simulink library "EHP_lib"  (Simulink 7.4)
settings: Solver=FixedStepDiscrete  StartTime=0.0  StopTime=Inf  FixedStep=0.001  RelTol=1e-3
values from neighbouring files (symbols this model uses):
  EHPc_BatIsoTestCmd = mpt.Parameter    [EHP_CAL.m]
  EHPc_r_ClcnRo = mpt.Parameter    [EHP_CAL.m]
  EHPc_r_IsoDiagInitVal = mpt.Parameter    [EHP_CAL.m]
undefined symbols (not defined in the file or in its folder): BCU_Drive_St, BCU_FastCharge_St, BCU_SlowCharge_St
libraries: Defined_Functionality x12, simulink x4
settings Model: Creator=yanlijuan2  LastModifiedBy=sunsijun

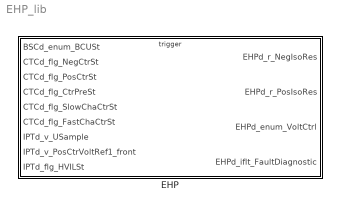
== system EHP_lib ==
  EHP : Subsystem  TreatAsAtomicUnit=on

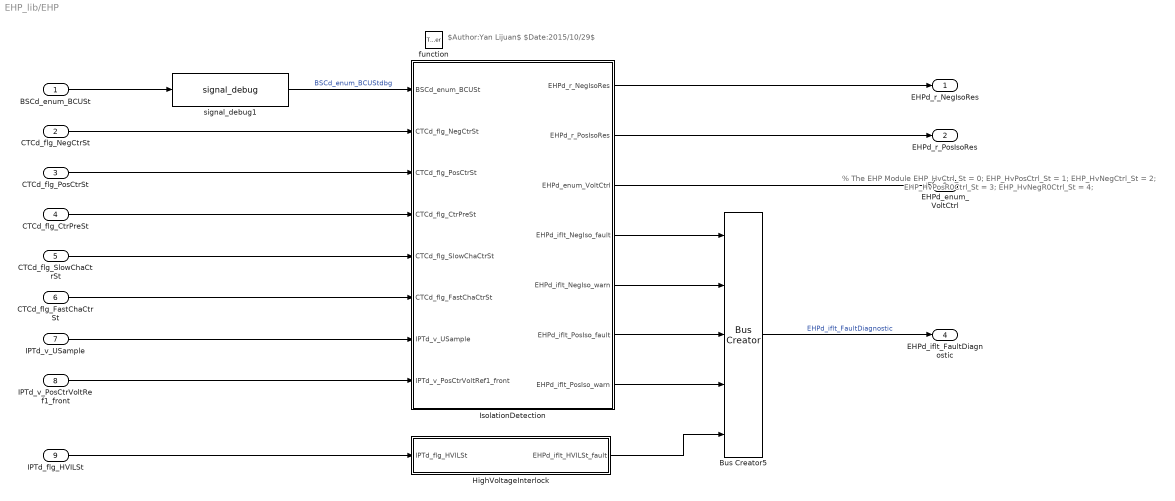
== system EHP_lib/EHP ==
  note: % The EHP Module
      | EHP_HvCtrl_St                       = 0;
      | EHP_HvPosCtrl_St                 = 1;
      | EHP_HvNegCtrl_St                 = 2;
      | EHP_HvPosR0Ctrl_St             = 3;
      | EHP_HvNegR0Ctrl_St             = 4;
  note: $Author:Yan Lijuan$
      | $Date:2015/10/29$
  BSCd_enum_BCUSt : Inport
  CTCd_flg_NegCtrSt : Inport  Port=2  OutDataType=fixdt(1, 16)  OutScaling=2^0
  CTCd_flg_PosCtrSt : Inport  Port=3  OutDataType=fixdt(1, 16)  OutScaling=2^0
  CTCd_flg_CtrPreSt : Inport  Port=4  OutDataType=fixdt(1, 16)  OutScaling=2^0
  CTCd_flg_SlowChaCtrSt : Inport  Port=5  OutDataType=fixdt(1, 16)  OutScaling=2^0
  CTCd_flg_FastChaCtrSt : Inport  Port=6  OutDataType=fixdt(1, 16)  OutScaling=2^0
  IPTd_v_USample : Inport  Port=7  OutDataType=fixdt(1, 16)  OutScaling=2^0
  IPTd_v_PosCtrVoltRef1_front : Inport  Port=8  OutDataType=fixdt(1, 16)  OutScaling=2^0
  IPTd_flg_HVILSt : Inport  Port=9  OutDataType=fixdt(1, 16)  OutScaling=2^0
  function : TriggerPort  TriggerType=function-call
  Bus Creator5 : BusCreator  Inputs=5
  HighVoltageInterlock : Subsystem  RTWFcnName=HighVoltageInterlock
      settings: RTWSystemCode=Function  RTWFcnNameOpts=User specified  RTWFileNameOpts=Use function name
  IsolationDetection : Subsystem  Description=|
      | $Author:Yan LiJuan$
      | $Date:2015/03/26$  
      | $Revision:1.0$
  signal_debug1 : Defined_Functionality/signal_debug  SystemSampleTime=-1  debug_switch=BSCc_dbgsw_BSCSt  debug_value=BSCc_dbgval_BSCSt
      settings: AttributesFormatString=[SWITCH=%<debug_switch>]\n[VALUE=%<debug_value>]
  EHPd_r_NegIsoRes : Outport  OutDataType=fixdt(1, 16)  OutScaling=2^0
  EHPd_r_PosIsoRes : Outport  Port=2  OutDataType=fixdt(1, 16)  OutScaling=2^0
  EHPd_enum_VoltCtrl : Outport  Port=3  OutDataType=fixdt(1, 16)  OutScaling=2^0
  EHPd_iflt_FaultDiagnostic : Outport  Port=4  OutDataType=fixdt(1, 16)  OutScaling=2^0
  wires:
  IPTd_v_PosCtrVoltRef1_front/1 -> IsolationDetection/8(IPTd_v_PosCtrVoltRef1_front)
  signal_debug1/1 -> IsolationDetection/1(BSCd_enum_BCUSt)  "BSCd_enum_BCUStdbg"
  IsolationDetection/3(EHPd_enum_VoltCtrl) -> EHPd_enum_VoltCtrl/1
  IsolationDetection/2(EHPd_r_PosIsoRes) -> EHPd_r_PosIsoRes/1
  IsolationDetection/1(EHPd_r_NegIsoRes) -> EHPd_r_NegIsoRes/1
  IPTd_flg_HVILSt/1 -> HighVoltageInterlock/1(IPTd_flg_HVILSt)
  HighVoltageInterlock/1(EHPd_iflt_HVILSt_fault) -> Bus Creator5/5
  IPTd_v_USample/1 -> IsolationDetection/7(IPTd_v_USample)
  CTCd_flg_CtrPreSt/1 -> IsolationDetection/4(CTCd_flg_CtrPreSt)
  CTCd_flg_PosCtrSt/1 -> IsolationDetection/3(CTCd_flg_PosCtrSt)
  CTCd_flg_NegCtrSt/1 -> IsolationDetection/2(CTCd_flg_NegCtrSt)
  IsolationDetection/4(EHPd_iflt_NegIso_fault) -> Bus Creator5/1
  IsolationDetection/5(EHPd_iflt_NegIso_warn) -> Bus Creator5/2
  IsolationDetection/6(EHPd_iflt_PosIso_fault) -> Bus Creator5/3
  IsolationDetection/7(EHPd_iflt_PosIso_warn) -> Bus Creator5/4
  Bus Creator5/1 -> EHPd_iflt_FaultDiagnostic/1  "EHPd_iflt_FaultDiagnostic"
  CTCd_flg_SlowChaCtrSt/1 -> IsolationDetection/5(CTCd_flg_SlowChaCtrSt)
  CTCd_flg_FastChaCtrSt/1 -> IsolationDetection/6(CTCd_flg_FastChaCtrSt)
  BSCd_enum_BCUSt/1 -> signal_debug1/1

== system EHP_lib/EHP/HighVoltageInterlock ==
  IPTd_flg_HVILSt : Inport  OutDataType=fixdt(1, 16)  OutScaling=2^0
  Gain : Gain  ParameterDataType=fixdt(1, 16)  ParameterScaling=2^0  OutDataType=fixdt(1, 16)  OutScaling=2^0  OutDataTypeStr=Inherit: Same as input
  EHPd_iflt_HVILSt_fault : Outport  OutDataType=fixdt(1, 16)  OutScaling=2^0
  wires:
  Gain/1 -> EHPd_iflt_HVILSt_fault/1  "EHPd_iflt_HVILSt_fault"
  IPTd_flg_HVILSt/1 -> Gain/1

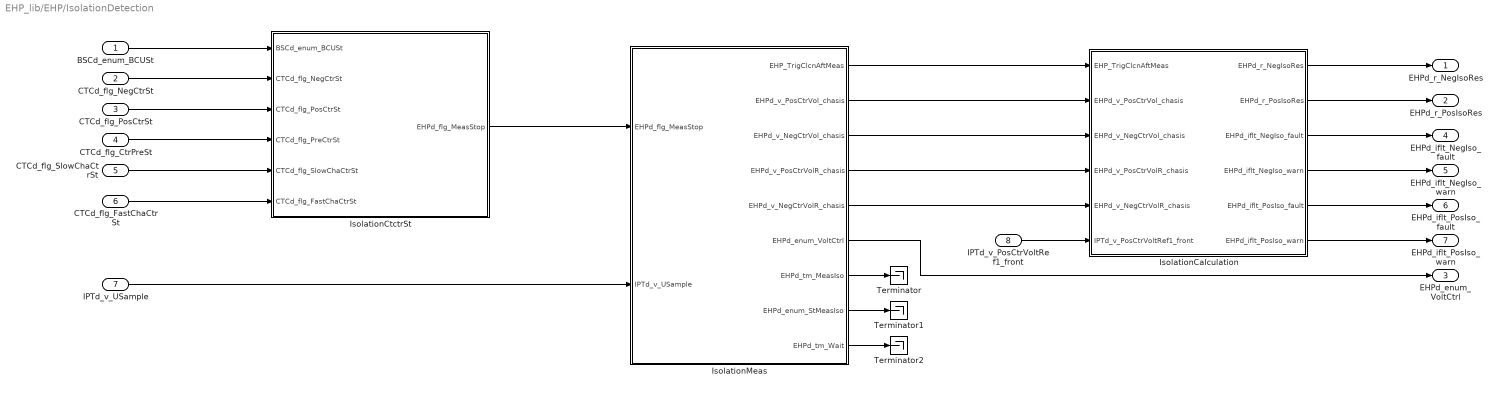
== system EHP_lib/EHP/IsolationDetection ==
  BSCd_enum_BCUSt : Inport
  CTCd_flg_NegCtrSt : Inport  Port=2  OutDataType=fixdt(1, 16)  OutScaling=2^0
  CTCd_flg_PosCtrSt : Inport  Port=3  OutDataType=fixdt(1, 16)  OutScaling=2^0
  CTCd_flg_CtrPreSt : Inport  Port=4  OutDataType=fixdt(1, 16)  OutScaling=2^0
  CTCd_flg_SlowChaCtrSt : Inport  Port=5  OutDataType=fixdt(1, 16)  OutScaling=2^0
  CTCd_flg_FastChaCtrSt : Inport  Port=6  OutDataType=fixdt(1, 16)  OutScaling=2^0
  IPTd_v_USample : Inport  Port=7  OutDataType=fixdt(1, 16)  OutScaling=2^0
  IPTd_v_PosCtrVoltRef1_front : Inport  Port=8  OutDataType=fixdt(1, 16)  OutScaling=2^0
  IsolationCalculation : Subsystem  Description=|
      | $Author:Yan LiJuan$
      | $Date:2015/03/26$  
      | $Revision:1.0$
  IsolationCtctrSt : Subsystem  Description=|
      | $Author:Yan LiJuan$
      | $Date:2015/06/03$  
      | $Revision:1.0$
  IsolationMeas : Subsystem  Description=|
      | $Author:Yan LiJuan$
      | $Date:2015/03/26$  
      | $Revision:1.0$
  Terminator : Terminator
  Terminator1 : Terminator
  Terminator2 : Terminator
  EHPd_r_NegIsoRes : Outport  OutDataType=fixdt(1, 16)  OutScaling=2^0
  EHPd_r_PosIsoRes : Outport  Port=2  OutDataType=fixdt(1, 16)  OutScaling=2^0
  EHPd_enum_VoltCtrl : Outport  Port=3  OutDataType=fixdt(1, 16)  OutScaling=2^0
  EHPd_iflt_NegIso_fault : Outport  Port=4  OutDataType=fixdt(1, 16)  OutScaling=2^0
  EHPd_iflt_NegIso_warn : Outport  Port=5  OutDataType=fixdt(1, 16)  OutScaling=2^0
  EHPd_iflt_PosIso_fault : Outport  Port=6  OutDataType=fixdt(1, 16)  OutScaling=2^0
  EHPd_iflt_PosIso_warn : Outport  Port=7  OutDataType=fixdt(1, 16)  OutScaling=2^0
  wires:
  IsolationMeas/9(EHPd_tm_Wait) -> Terminator2/1
  IsolationMeas/8(EHPd_enum_StMeasIso) -> Terminator1/1
  IsolationMeas/7(EHPd_tm_MeasIso) -> Terminator/1
  IPTd_v_PosCtrVoltRef1_front/1 -> IsolationCalculation/6(IPTd_v_PosCtrVoltRef1_front)
  IsolationMeas/6(EHPd_enum_VoltCtrl) -> EHPd_enum_VoltCtrl/1
  IsolationCalculation/6(EHPd_iflt_PosIso_warn) -> EHPd_iflt_PosIso_warn/1
  IsolationCalculation/5(EHPd_iflt_PosIso_fault) -> EHPd_iflt_PosIso_fault/1
  IsolationCalculation/4(EHPd_iflt_NegIso_warn) -> EHPd_iflt_NegIso_warn/1
  IsolationCalculation/3(EHPd_iflt_NegIso_fault) -> EHPd_iflt_NegIso_fault/1
  IsolationCalculation/2(EHPd_r_PosIsoRes) -> EHPd_r_PosIsoRes/1
  IsolationCalculation/1(EHPd_r_NegIsoRes) -> EHPd_r_NegIsoRes/1
  IsolationMeas/4(EHPd_v_PosCtrVolR_chasis) -> IsolationCalculation/4(EHPd_v_PosCtrVolR_chasis)
  IsolationMeas/1(EHP_TrigClcnAftMeas) -> IsolationCalculation/1(EHP_TrigClcnAftMeas)
  CTCd_flg_CtrPreSt/1 -> IsolationCtctrSt/4(CTCd_flg_PreCtrSt)
  CTCd_flg_PosCtrSt/1 -> IsolationCtctrSt/3(CTCd_flg_PosCtrSt)
  CTCd_flg_NegCtrSt/1 -> IsolationCtctrSt/2(CTCd_flg_NegCtrSt)
  IsolationMeas/5(EHPd_v_NegCtrVolR_chasis) -> IsolationCalculation/5(EHPd_v_NegCtrVolR_chasis)
  IPTd_v_USample/1 -> IsolationMeas/2(IPTd_v_USample)
  IsolationMeas/3(EHPd_v_NegCtrVol_chasis) -> IsolationCalculation/3(EHPd_v_NegCtrVol_chasis)
  IsolationCtctrSt/1(EHPd_flg_MeasStop) -> IsolationMeas/1(EHPd_flg_MeasStop)
  IsolationMeas/2(EHPd_v_PosCtrVol_chasis) -> IsolationCalculation/2(EHPd_v_PosCtrVol_chasis)
  CTCd_flg_SlowChaCtrSt/1 -> IsolationCtctrSt/5(CTCd_flg_SlowChaCtrSt)
  CTCd_flg_FastChaCtrSt/1 -> IsolationCtctrSt/6(CTCd_flg_FastChaCtrSt)
  BSCd_enum_BCUSt/1 -> IsolationCtctrSt/1(BSCd_enum_BCUSt)

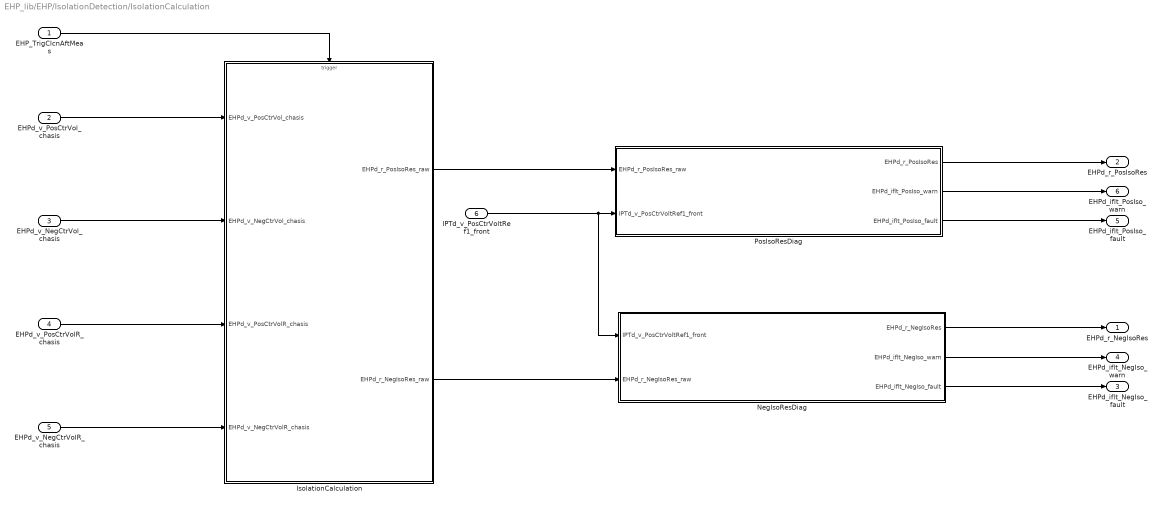
== system EHP_lib/EHP/IsolationDetection/IsolationCalculation ==
  EHP_TrigClcnAftMeas : Inport  OutDataType=fixdt(1, 16)  OutScaling=2^0
  EHPd_v_PosCtrVol_chasis : Inport  Port=2  OutDataType=fixdt(1, 16)  OutScaling=2^0
  EHPd_v_NegCtrVol_chasis : Inport  Port=3  OutDataType=fixdt(1, 16)  OutScaling=2^0
  EHPd_v_PosCtrVolR_chasis : Inport  Port=4  OutDataType=fixdt(1, 16)  OutScaling=2^0
  EHPd_v_NegCtrVolR_chasis : Inport  Port=5  OutDataType=fixdt(1, 16)  OutScaling=2^0
  IPTd_v_PosCtrVoltRef1_front : Inport  Port=6  OutDataType=fixdt(1, 16)  OutScaling=2^0
  IsolationCalculation : Subsystem  Description=|
      | $Author:Yan LiJuan$
      | $Date:2015/03/26$  
      | $Revision:1.0$
  NegIsoResDiag : Subsystem
  PosIsoResDiag : Subsystem
  EHPd_r_NegIsoRes : Outport  OutDataType=fixdt(1, 16)  OutScaling=2^0
  EHPd_r_PosIsoRes : Outport  Port=2  OutDataType=fixdt(1, 16)  OutScaling=2^0
  EHPd_iflt_NegIso_fault : Outport  Port=3  OutDataType=fixdt(1, 16)  OutScaling=2^0
  EHPd_iflt_NegIso_warn : Outport  Port=4  OutDataType=fixdt(1, 16)  OutScaling=2^0
  EHPd_iflt_PosIso_fault : Outport  Port=5  OutDataType=fixdt(1, 16)  OutScaling=2^0
  EHPd_iflt_PosIso_warn : Outport  Port=6  OutDataType=fixdt(1, 16)  OutScaling=2^0
  wires:
  NegIsoResDiag/3(EHPd_iflt_NegIso_fault) -> EHPd_iflt_NegIso_fault/1
  NegIsoResDiag/2(EHPd_iflt_NegIso_warn) -> EHPd_iflt_NegIso_warn/1
  NegIsoResDiag/1(EHPd_r_NegIsoRes) -> EHPd_r_NegIsoRes/1
  IsolationCalculation/2(EHPd_r_NegIsoRes_raw) -> NegIsoResDiag/2(EHPd_r_NegIsoRes_raw)
  PosIsoResDiag/3(EHPd_iflt_PosIso_fault) -> EHPd_iflt_PosIso_fault/1
  PosIsoResDiag/2(EHPd_iflt_PosIso_warn) -> EHPd_iflt_PosIso_warn/1
  PosIsoResDiag/1(EHPd_r_PosIsoRes) -> EHPd_r_PosIsoRes/1
  IPTd_v_PosCtrVoltRef1_front/1 -> NegIsoResDiag/1(IPTd_v_PosCtrVoltRef1_front), PosIsoResDiag/2(IPTd_v_PosCtrVoltRef1_front)
  EHPd_v_NegCtrVolR_chasis/1 -> IsolationCalculation/4(EHPd_v_NegCtrVolR_chasis)
  EHPd_v_PosCtrVolR_chasis/1 -> IsolationCalculation/3(EHPd_v_PosCtrVolR_chasis)
  EHPd_v_NegCtrVol_chasis/1 -> IsolationCalculation/2(EHPd_v_NegCtrVol_chasis)
  EHPd_v_PosCtrVol_chasis/1 -> IsolationCalculation/1(EHPd_v_PosCtrVol_chasis)
  IsolationCalculation/1(EHPd_r_PosIsoRes_raw) -> PosIsoResDiag/1(EHPd_r_PosIsoRes_raw)
  EHP_TrigClcnAftMeas/1 -> IsolationCalculation/Trigger

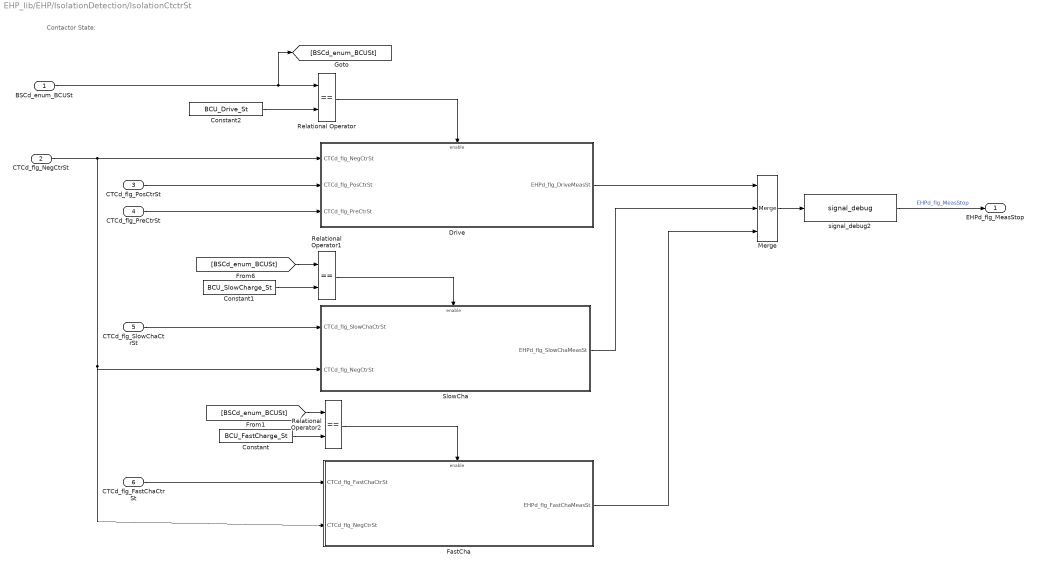
== system EHP_lib/EHP/IsolationDetection/IsolationCtctrSt ==
  note: Contactor State:
  BSCd_enum_BCUSt : Inport
  CTCd_flg_NegCtrSt : Inport  Port=2  OutDataType=fixdt(1, 16)  OutScaling=2^0
  CTCd_flg_PosCtrSt : Inport  Port=3  OutDataType=fixdt(1, 16)  OutScaling=2^0
  CTCd_flg_PreCtrSt : Inport  Port=4  OutDataType=fixdt(1, 16)  OutScaling=2^0
  CTCd_flg_SlowChaCtrSt : Inport  Port=5  OutDataType=fixdt(1, 16)  OutScaling=2^0
  CTCd_flg_FastChaCtrSt : Inport  Port=6  OutDataType=fixdt(1, 16)  OutScaling=2^0
  Constant : Constant  Value=BCU_FastCharge_St  OutDataTypeMode=uint8  OutDataType=fixdt(1, 16)  OutScaling=2^0  OutDataTypeStr=uint8
  Constant1 : Constant  Value=BCU_SlowCharge_St  OutDataTypeMode=uint8  OutDataType=fixdt(1, 16)  OutScaling=2^0  OutDataTypeStr=uint8
  Constant2 : Constant  Value=BCU_Drive_St  OutDataTypeMode=uint8  OutDataType=fixdt(1, 16)  OutScaling=2^0  OutDataTypeStr=uint8
  Drive : Subsystem  Description=|
      | $Author:Yan LiJuan$
      | $Date:2015/06/03$  
      | $Revision:1.0$
  FastCha : Subsystem  Description=|
      | $Author:Yan LiJuan$
      | $Date:2015/06/03$  
      | $Revision:1.0$
  Merge : Merge  Inputs=3
  Relational Operator : RelationalOperator  Operator===  LogicOutDataTypeMode=boolean  LogicDataType=fixdt(0, 8)  OutDataTypeStr=boolean
  Relational Operator1 : RelationalOperator  Operator===  LogicOutDataTypeMode=boolean  LogicDataType=fixdt(0, 8)  OutDataTypeStr=boolean
  Relational Operator2 : RelationalOperator  Operator===  LogicOutDataTypeMode=boolean  LogicDataType=fixdt(0, 8)  OutDataTypeStr=boolean
  SlowCha : Subsystem  Description=|
      | $Author:Yan LiJuan$
      | $Date:2015/06/03$  
      | $Revision:1.0$
  signal_debug2 : Defined_Functionality/signal_debug  SystemSampleTime=-1  debug_switch=EHPc_dbgsw_MeasStop  debug_value=EHPc_dbgval_MeasStop
      settings: AttributesFormatString=[SWITCH=%<debug_switch>]\n[VALUE=%<debug_value>]
  EHPd_flg_MeasStop : Outport  OutDataType=fixdt(1, 16)  OutScaling=2^0
  wires:
  signal_debug2/1 -> EHPd_flg_MeasStop/1  "EHPd_flg_MeasStop"
  CTCd_flg_PreCtrSt/1 -> Drive/3(CTCd_flg_PreCtrSt)
  CTCd_flg_SlowChaCtrSt/1 -> SlowCha/1(CTCd_flg_SlowChaCtrSt)
  Drive/1(EHPd_flg_DriveMeasSt) -> Merge/1
  SlowCha/1(EHPd_flg_SlowChaMeasSt) -> Merge/2
  FastCha/1(EHPd_flg_FastChaMeasSt) -> Merge/3
  Merge/1 -> signal_debug2/1
  Constant1/1 -> Relational Operator1/2
  [BSCd_enum_BCUSt] -> Relational Operator1/1
  Relational Operator1/1 -> SlowCha/Enable
  CTCd_flg_NegCtrSt/1 -> Drive/1(CTCd_flg_NegCtrSt), SlowCha/2(CTCd_flg_NegCtrSt), FastCha/2(CTCd_flg_NegCtrSt)
  CTCd_flg_PosCtrSt/1 -> Drive/2(CTCd_flg_PosCtrSt)
  CTCd_flg_FastChaCtrSt/1 -> FastCha/1(CTCd_flg_FastChaCtrSt)
  BSCd_enum_BCUSt/1 -> Relational Operator/1, [BSCd_enum_BCUSt]
  Constant2/1 -> Relational Operator/2
  Relational Operator/1 -> Drive/Enable
  Constant/1 -> Relational Operator2/2
  [BSCd_enum_BCUSt] -> Relational Operator2/1
  Relational Operator2/1 -> FastCha/Enable

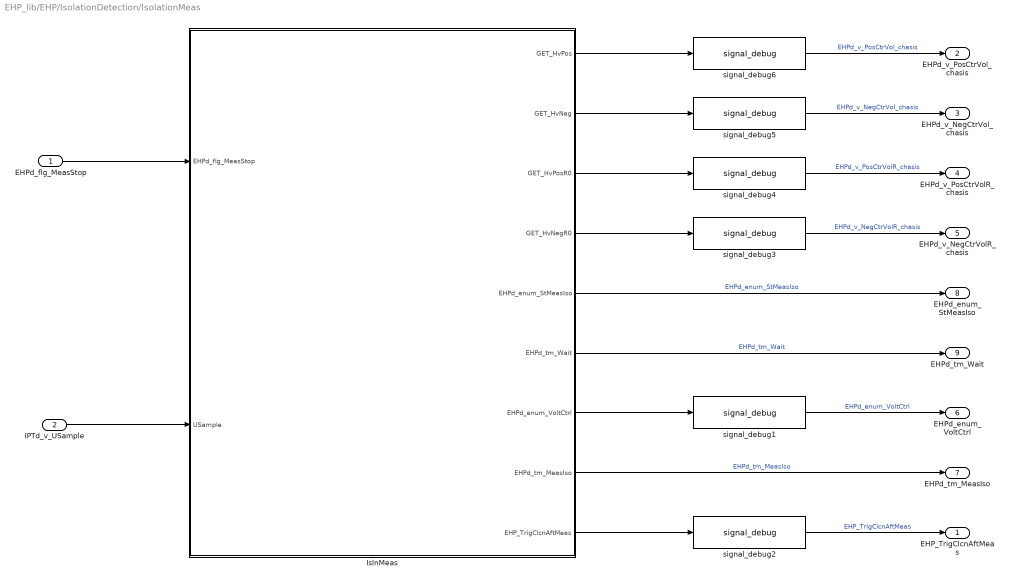
== system EHP_lib/EHP/IsolationDetection/IsolationMeas ==
  EHPd_flg_MeasStop : Inport  DataType=boolean  OutDataType=fixdt(1, 16)  OutScaling=2^0  OutDataTypeStr=boolean
  IPTd_v_USample : Inport  Port=2  OutDataType=fixdt(1, 16)  OutScaling=2^0
  IslnMeas : Stateflow chart  Description=|
      | $Author:Yan LiJuan$
      | $Date:2015/03/26$  
      | $Revision:1.0$
  signal_debug1 : Defined_Functionality/signal_debug  SystemSampleTime=-1  debug_switch=EHPc_dbgsw_VoltCtrl  debug_value=EHPc_dbgval_VoltCtrl
      settings: AttributesFormatString=[SWITCH=%<debug_switch>]\n[VALUE=%<debug_value>]
  signal_debug2 : Defined_Functionality/signal_debug  SystemSampleTime=-1  debug_switch=EHPc_dbgsw_TrigClcnAftMeas  debug_value=EHPc_dbgval_TrigClcnAftMeas
      settings: AttributesFormatString=[SWITCH=%<debug_switch>]\n[VALUE=%<debug_value>]
  signal_debug3 : Defined_Functionality/signal_debug  SystemSampleTime=-1  debug_switch=IPTc_dbgsw_NegCtrVolR  debug_value=IPTc_dbgval_NegCtrVolR
      settings: AttributesFormatString=[SWITCH=%<debug_switch>]\n[VALUE=%<debug_value>]
  signal_debug4 : Defined_Functionality/signal_debug  SystemSampleTime=-1  debug_switch=IPTc_dbgsw_PosCtrVolR  debug_value=IPTc_dbgval_PosCtrVolR
      settings: AttributesFormatString=[SWITCH=%<debug_switch>]\n[VALUE=%<debug_value>]
  signal_debug5 : Defined_Functionality/signal_debug  SystemSampleTime=-1  debug_switch=IPTc_dbgsw_NegCtrVol  debug_value=IPTc_dbgval_NegCtrVol
      settings: AttributesFormatString=[SWITCH=%<debug_switch>]\n[VALUE=%<debug_value>]
  signal_debug6 : Defined_Functionality/signal_debug  SystemSampleTime=-1  debug_switch=IPTc_dbgsw_PosCtrVol  debug_value=IPTc_dbgval_PosCtrVol
      settings: AttributesFormatString=[SWITCH=%<debug_switch>]\n[VALUE=%<debug_value>]
  EHP_TrigClcnAftMeas : Outport  OutDataType=fixdt(1, 16)  OutScaling=2^0
  EHPd_v_PosCtrVol_chasis : Outport  Port=2  OutDataType=fixdt(1, 16)  OutScaling=2^0
  EHPd_v_NegCtrVol_chasis : Outport  Port=3  OutDataType=fixdt(1, 16)  OutScaling=2^0
  EHPd_v_PosCtrVolR_chasis : Outport  Port=4  OutDataType=fixdt(1, 16)  OutScaling=2^0
  EHPd_v_NegCtrVolR_chasis : Outport  Port=5  OutDataType=fixdt(1, 16)  OutScaling=2^0
  EHPd_enum_VoltCtrl : Outport  Port=6  OutDataType=fixdt(1, 16)  OutScaling=2^0
  EHPd_tm_MeasIso : Outport  Port=7  OutDataType=fixdt(1, 16)  OutScaling=2^0
  EHPd_enum_StMeasIso : Outport  Port=8  OutDataType=fixdt(1, 16)  OutScaling=2^0
  EHPd_tm_Wait : Outport  Port=9  OutDataType=fixdt(1, 16)  OutScaling=2^0
  wires:
  IslnMeas/6(EHPd_tm_Wait) -> EHPd_tm_Wait/1  "EHPd_tm_Wait"
  IslnMeas/5(EHPd_enum_StMeasIso) -> EHPd_enum_StMeasIso/1  "EHPd_enum_StMeasIso"
  IslnMeas/8(EHPd_tm_MeasIso) -> EHPd_tm_MeasIso/1  "EHPd_tm_MeasIso"
  signal_debug6/1 -> EHPd_v_PosCtrVol_chasis/1  "EHPd_v_PosCtrVol_chasis"
  signal_debug5/1 -> EHPd_v_NegCtrVol_chasis/1  "EHPd_v_NegCtrVol_chasis"
  signal_debug4/1 -> EHPd_v_PosCtrVolR_chasis/1  "EHPd_v_PosCtrVolR_chasis"
  signal_debug3/1 -> EHPd_v_NegCtrVolR_chasis/1  "EHPd_v_NegCtrVolR_chasis"
  signal_debug2/1 -> EHP_TrigClcnAftMeas/1  "EHP_TrigClcnAftMeas"
  signal_debug1/1 -> EHPd_enum_VoltCtrl/1  "EHPd_enum_VoltCtrl"
  IslnMeas/7(EHPd_enum_VoltCtrl) -> signal_debug1/1
  EHPd_flg_MeasStop/1 -> IslnMeas/1(EHPd_flg_MeasStop)
  IslnMeas/9(EHP_TrigClcnAftMeas) -> signal_debug2/1
  IslnMeas/4(GET_HvNegR0) -> signal_debug3/1
  IslnMeas/3(GET_HvPosR0) -> signal_debug4/1
  IslnMeas/2(GET_HvNeg) -> signal_debug5/1
  IslnMeas/1(GET_HvPos) -> signal_debug6/1
  IPTd_v_USample/1 -> IslnMeas/2(USample)

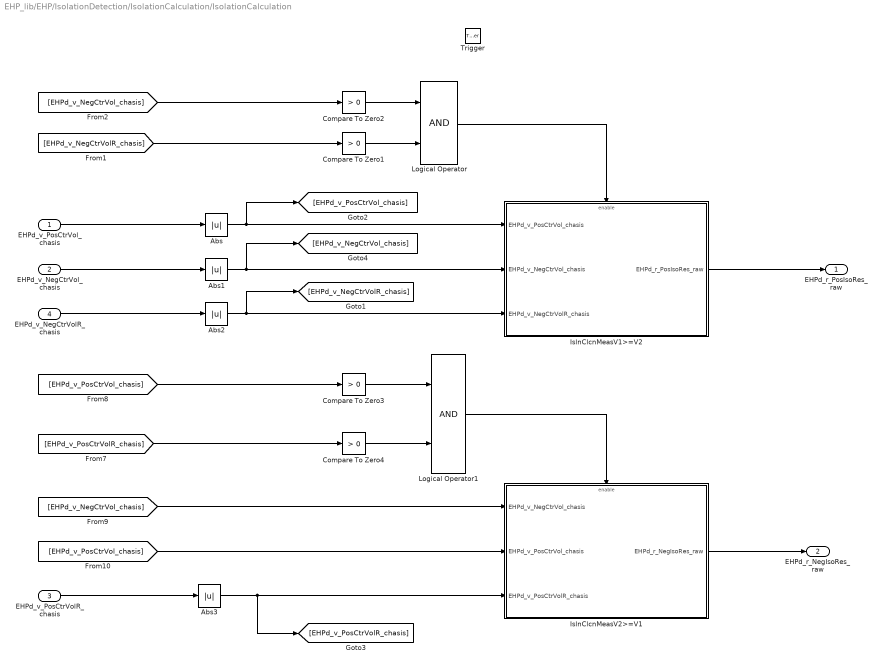
== system EHP_lib/EHP/IsolationDetection/IsolationCalculation/IsolationCalculation ==
  EHPd_v_PosCtrVol_chasis : Inport  OutDataType=fixdt(1, 16)  OutScaling=2^0
  EHPd_v_NegCtrVol_chasis : Inport  Port=2  OutDataType=fixdt(1, 16)  OutScaling=2^0
  EHPd_v_PosCtrVolR_chasis : Inport  Port=3  OutDataType=fixdt(1, 16)  OutScaling=2^0
  EHPd_v_NegCtrVolR_chasis : Inport  Port=4  OutDataType=fixdt(1, 16)  OutScaling=2^0
  Trigger : TriggerPort
  Abs{,1..3} (4 alike) : Abs  OutDataType=fixdt(1, 16)  OutScaling=2^0
  Compare To Zero{1..4} (4 alike) : simulink/Logic and Bit Operations/Compare To Zero  SystemSampleTime=-1  relop=>  LogicOutDataTypeMode=uint8
  IslnClcnMeasV1>=V2 : Subsystem  TreatAsAtomicUnit=on
  IslnClcnMeasV2>=V1 : Subsystem  TreatAsAtomicUnit=on
  Logical Operator : Logic  AllPortsSameDT=off  OutDataTypeMode=boolean  LogicDataType=fixdt(0, 8)  OutDataTypeStr=boolean
  Logical Operator1 : Logic  AllPortsSameDT=off  OutDataTypeMode=boolean  LogicDataType=fixdt(0, 8)  OutDataTypeStr=boolean
  EHPd_r_PosIsoRes_raw : Outport  OutDataType=fixdt(1, 16)  OutScaling=2^0
  EHPd_r_NegIsoRes_raw : Outport  Port=2  OutDataType=fixdt(1, 16)  OutScaling=2^0
  wires:
  Abs3/1 -> [EHPd_v_PosCtrVolR_chasis], IslnClcnMeasV2>=V1/3(EHPd_v_PosCtrVolR_chasis)
  Abs2/1 -> [EHPd_v_NegCtrVolR_chasis], IslnClcnMeasV1>=V2/3(EHPd_v_NegCtrVolR_chasis)
  Abs1/1 -> [EHPd_v_NegCtrVol_chasis], IslnClcnMeasV1>=V2/2(EHPd_v_NegCtrVol_chasis)
  Abs/1 -> IslnClcnMeasV1>=V2/1(EHPd_v_PosCtrVol_chasis), [EHPd_v_PosCtrVol_chasis]
  Compare To Zero4/1 -> Logical Operator1/2
  Compare To Zero3/1 -> Logical Operator1/1
  Compare To Zero1/1 -> Logical Operator/2
  Compare To Zero2/1 -> Logical Operator/1
  Logical Operator1/1 -> IslnClcnMeasV2>=V1/Enable
  [EHPd_v_PosCtrVolR_chasis] -> Compare To Zero4/1
  [EHPd_v_PosCtrVol_chasis] -> Compare To Zero3/1
  IslnClcnMeasV2>=V1/1(EHPd_r_NegIsoRes_raw) -> EHPd_r_NegIsoRes_raw/1
  IslnClcnMeasV1>=V2/1(EHPd_r_PosIsoRes_raw) -> EHPd_r_PosIsoRes_raw/1
  [EHPd_v_NegCtrVolR_chasis] -> Compare To Zero1/1
  [EHPd_v_NegCtrVol_chasis] -> Compare To Zero2/1
  Logical Operator/1 -> IslnClcnMeasV1>=V2/Enable
  EHPd_v_PosCtrVolR_chasis/1 -> Abs3/1
  [EHPd_v_PosCtrVol_chasis] -> IslnClcnMeasV2>=V1/2(EHPd_v_PosCtrVol_chasis)
  [EHPd_v_NegCtrVol_chasis] -> IslnClcnMeasV2>=V1/1(EHPd_v_NegCtrVol_chasis)
  EHPd_v_NegCtrVolR_chasis/1 -> Abs2/1
  EHPd_v_PosCtrVol_chasis/1 -> Abs/1
  EHPd_v_NegCtrVol_chasis/1 -> Abs1/1

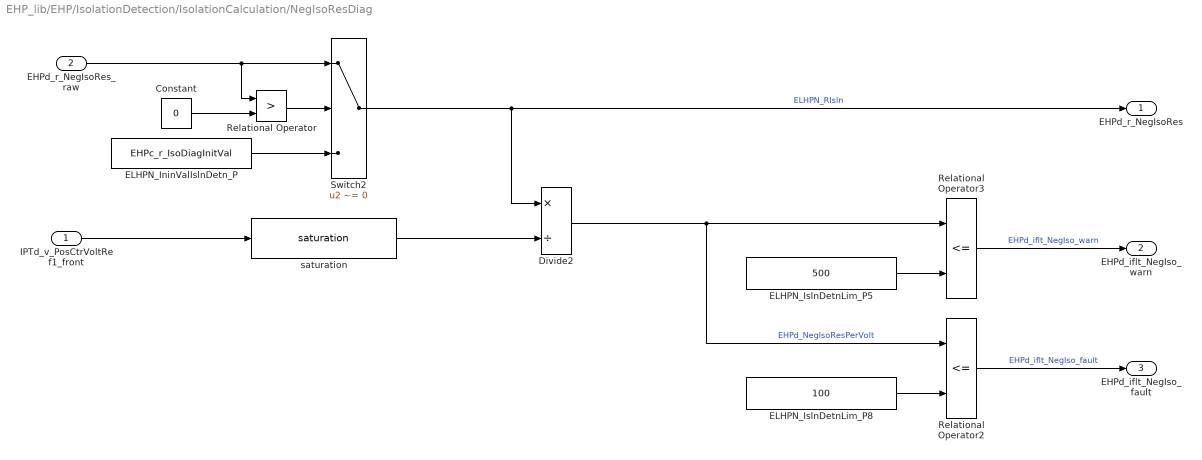
== system EHP_lib/EHP/IsolationDetection/IsolationCalculation/NegIsoResDiag ==
  IPTd_v_PosCtrVoltRef1_front : Inport  OutDataType=fixdt(1, 16)  OutScaling=2^0
  EHPd_r_NegIsoRes_raw : Inport  Port=2  OutDataType=fixdt(1, 16)  OutScaling=2^0
  Constant : Constant  Value=0  OutDataType=fixdt(1, 16)  OutScaling=2^0
  Divide2 : Product  Inputs=*/  OutDataType=fixdt(1, 16)  OutScaling=2^-10
  ELHPN_IninValIslnDetn_P : Constant  Value=EHPc_r_IsoDiagInitVal  OutDataType=fixdt(1, 16)  OutScaling=2^0
  ELHPN_IslnDetnLim_P5 : Constant  Value=500  OutDataTypeMode=single  OutDataType=fixdt(1, 16)  OutScaling=2^0  OutDataTypeStr=single
  ELHPN_IslnDetnLim_P8 : Constant  Value=100  OutDataTypeMode=single  OutDataType=fixdt(1, 16)  OutScaling=2^0  OutDataTypeStr=single
  Relational Operator : RelationalOperator  Operator=>  LogicOutDataTypeMode=boolean  LogicDataType=fixdt(0, 8)  OutDataTypeStr=boolean
  Relational Operator2 : RelationalOperator  Operator=<=  LogicOutDataTypeMode=boolean  LogicDataType=fixdt(0, 8)  OutDataTypeStr=boolean
  Relational Operator3 : RelationalOperator  Operator=<=  LogicOutDataTypeMode=boolean  LogicDataType=fixdt(0, 8)  OutDataTypeStr=boolean
  Switch2 : Switch  Criteria=u2 ~= 0  OutDataType=fixdt(1, 16)  OutScaling=2^0
  saturation : Defined_Functionality/saturation  SystemSampleTime=-1  upper_limit=800  lower_limit=10
      settings: AttributesFormatString=[UPPER_LIMIT=%<upper_limit>]\n[LOWER_LIMIT=%<lower_limit>]
  EHPd_r_NegIsoRes : Outport  OutDataType=fixdt(1, 16)  OutScaling=2^0
  EHPd_iflt_NegIso_warn : Outport  Port=2  OutDataType=fixdt(1, 16)  OutScaling=2^0
  EHPd_iflt_NegIso_fault : Outport  Port=3  OutDataType=fixdt(1, 16)  OutScaling=2^0
  wires:
  ELHPN_IninValIslnDetn_P/1 -> Switch2/3
  Relational Operator/1 -> Switch2/2
  Constant/1 -> Relational Operator/2
  saturation/1 -> Divide2/2
  IPTd_v_PosCtrVoltRef1_front/1 -> saturation/1
  ELHPN_IslnDetnLim_P8/1 -> Relational Operator2/2
  Divide2/1 -> Relational Operator2/1, Relational Operator3/1  "EHPd_NegIsoResPerVolt"
  ELHPN_IslnDetnLim_P5/1 -> Relational Operator3/2
  EHPd_r_NegIsoRes_raw/1 -> Switch2/1, Relational Operator/1
  Relational Operator3/1 -> EHPd_iflt_NegIso_warn/1  "EHPd_iflt_NegIso_warn"
  Relational Operator2/1 -> EHPd_iflt_NegIso_fault/1  "EHPd_iflt_NegIso_fault"
  Switch2/1 -> Divide2/1, EHPd_r_NegIsoRes/1  "ELHPN_RIsln"

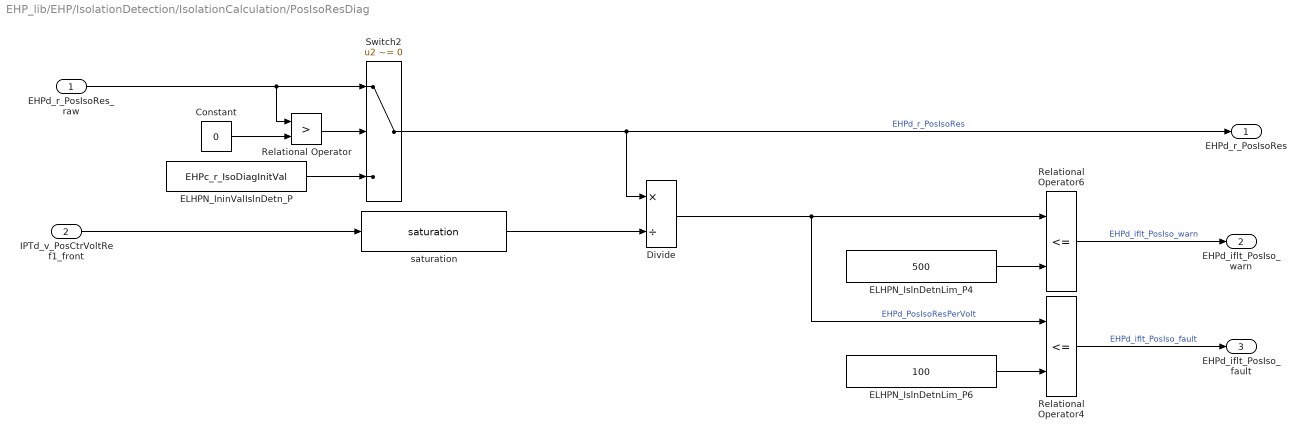
== system EHP_lib/EHP/IsolationDetection/IsolationCalculation/PosIsoResDiag ==
  EHPd_r_PosIsoRes_raw : Inport  OutDataType=fixdt(1, 16)  OutScaling=2^0
  IPTd_v_PosCtrVoltRef1_front : Inport  Port=2  OutDataType=fixdt(1, 16)  OutScaling=2^0
  Constant : Constant  Value=0  OutDataType=fixdt(1, 16)  OutScaling=2^0
  Divide : Product  Inputs=*/  OutDataType=fixdt(1, 16)  OutScaling=2^-10
  ELHPN_IninValIslnDetn_P : Constant  Value=EHPc_r_IsoDiagInitVal  OutDataType=fixdt(1, 16)  OutScaling=2^0
  ELHPN_IslnDetnLim_P4 : Constant  Value=500  OutDataTypeMode=single  OutDataType=fixdt(1, 16)  OutScaling=2^0  OutDataTypeStr=single
  ELHPN_IslnDetnLim_P6 : Constant  Value=100  OutDataTypeMode=single  OutDataType=fixdt(1, 16)  OutScaling=2^0  OutDataTypeStr=single
  Relational Operator : RelationalOperator  Operator=>  LogicOutDataTypeMode=boolean  LogicDataType=fixdt(0, 8)  OutDataTypeStr=boolean
  Relational Operator4 : RelationalOperator  Operator=<=  LogicOutDataTypeMode=boolean  LogicDataType=fixdt(0, 8)  OutDataTypeStr=boolean
  Relational Operator6 : RelationalOperator  Operator=<=  LogicOutDataTypeMode=boolean  LogicDataType=fixdt(0, 8)  OutDataTypeStr=boolean
  Switch2 : Switch  Criteria=u2 ~= 0  OutDataType=fixdt(1, 16)  OutScaling=2^0
  saturation : Defined_Functionality/saturation  SystemSampleTime=-1  upper_limit=800  lower_limit=10
      settings: AttributesFormatString=[UPPER_LIMIT=%<upper_limit>]\n[LOWER_LIMIT=%<lower_limit>]
  EHPd_r_PosIsoRes : Outport  OutDataType=fixdt(1, 16)  OutScaling=2^0
  EHPd_iflt_PosIso_warn : Outport  Port=2  OutDataType=fixdt(1, 16)  OutScaling=2^0
  EHPd_iflt_PosIso_fault : Outport  Port=3  OutDataType=fixdt(1, 16)  OutScaling=2^0
  wires:
  ELHPN_IninValIslnDetn_P/1 -> Switch2/3
  Relational Operator/1 -> Switch2/2
  Constant/1 -> Relational Operator/2
  EHPd_r_PosIsoRes_raw/1 -> Switch2/1, Relational Operator/1
  saturation/1 -> Divide/2
  Divide/1 -> Relational Operator4/1, Relational Operator6/1  "EHPd_PosIsoResPerVolt"
  ELHPN_IslnDetnLim_P6/1 -> Relational Operator4/2
  ELHPN_IslnDetnLim_P4/1 -> Relational Operator6/2
  IPTd_v_PosCtrVoltRef1_front/1 -> saturation/1
  Relational Operator6/1 -> EHPd_iflt_PosIso_warn/1  "EHPd_iflt_PosIso_warn"
  Relational Operator4/1 -> EHPd_iflt_PosIso_fault/1  "EHPd_iflt_PosIso_fault"
  Switch2/1 -> EHPd_r_PosIsoRes/1, Divide/1  "EHPd_r_PosIsoRes"

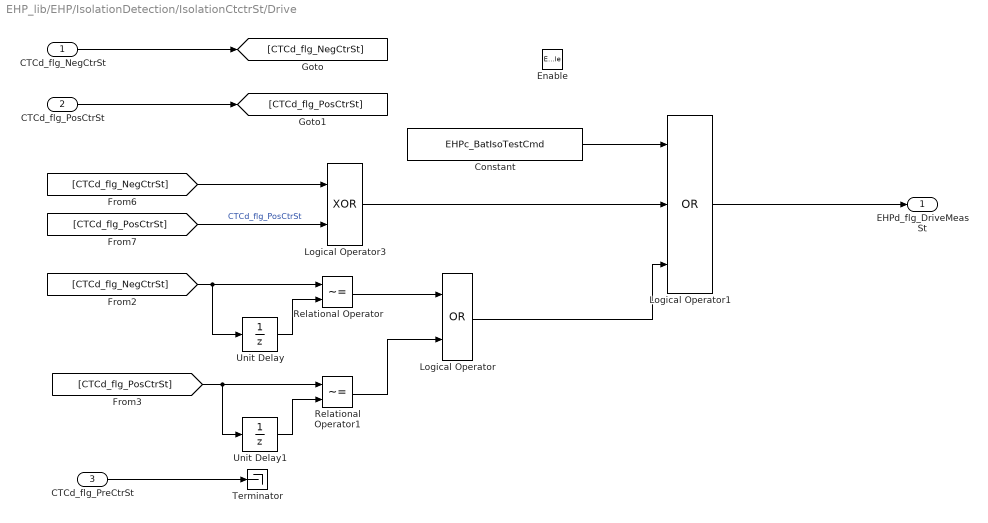
== system EHP_lib/EHP/IsolationDetection/IsolationCtctrSt/Drive ==
  CTCd_flg_NegCtrSt : Inport  OutDataType=fixdt(1, 16)  OutScaling=2^0
  CTCd_flg_PosCtrSt : Inport  Port=2  OutDataType=fixdt(1, 16)  OutScaling=2^0
  CTCd_flg_PreCtrSt : Inport  Port=3  OutDataType=fixdt(1, 16)  OutScaling=2^0
  Enable : EnablePort
  Constant : Constant  Value=EHPc_BatIsoTestCmd  OutDataTypeMode=boolean  OutDataType=fixdt(1, 16)  OutScaling=2^0  OutDataTypeStr=boolean
  Logical Operator : Logic  Operator=OR  AllPortsSameDT=off  OutDataTypeMode=boolean  LogicDataType=fixdt(0, 8)  OutDataTypeStr=boolean
  Logical Operator1 : Logic  Operator=OR  Inputs=3  AllPortsSameDT=off  OutDataTypeMode=boolean  LogicDataType=fixdt(0, 8)  OutDataTypeStr=boolean
  Logical Operator3 : Logic  Operator=XOR  AllPortsSameDT=off  OutDataTypeMode=boolean  LogicDataType=fixdt(0, 8)  OutDataTypeStr=boolean
  Relational Operator : RelationalOperator  Operator=~=  LogicOutDataTypeMode=boolean  LogicDataType=fixdt(0, 8)  OutDataTypeStr=boolean
  Relational Operator1 : RelationalOperator  Operator=~=  LogicOutDataTypeMode=boolean  LogicDataType=fixdt(0, 8)  OutDataTypeStr=boolean
  Terminator : Terminator
  Unit Delay : UnitDelay  SampleTime=-1
  Unit Delay1 : UnitDelay  SampleTime=-1
  EHPd_flg_DriveMeasSt : Outport  OutDataType=fixdt(1, 16)  OutScaling=2^0
  wires:
  Constant/1 -> Logical Operator1/1
  Logical Operator1/1 -> EHPd_flg_DriveMeasSt/1
  CTCd_flg_PreCtrSt/1 -> Terminator/1
  Logical Operator3/1 -> Logical Operator1/2
  Logical Operator/1 -> Logical Operator1/3
  [CTCd_flg_PosCtrSt] -> Logical Operator3/2  "CTCd_flg_PosCtrSt"
  [CTCd_flg_NegCtrSt] -> Logical Operator3/1
  Relational Operator1/1 -> Logical Operator/2
  Relational Operator/1 -> Logical Operator/1
  Unit Delay1/1 -> Relational Operator1/2
  [CTCd_flg_PosCtrSt] -> Unit Delay1/1, Relational Operator1/1
  Unit Delay/1 -> Relational Operator/2
  [CTCd_flg_NegCtrSt] -> Unit Delay/1, Relational Operator/1
  CTCd_flg_PosCtrSt/1 -> [CTCd_flg_PosCtrSt]
  CTCd_flg_NegCtrSt/1 -> [CTCd_flg_NegCtrSt]

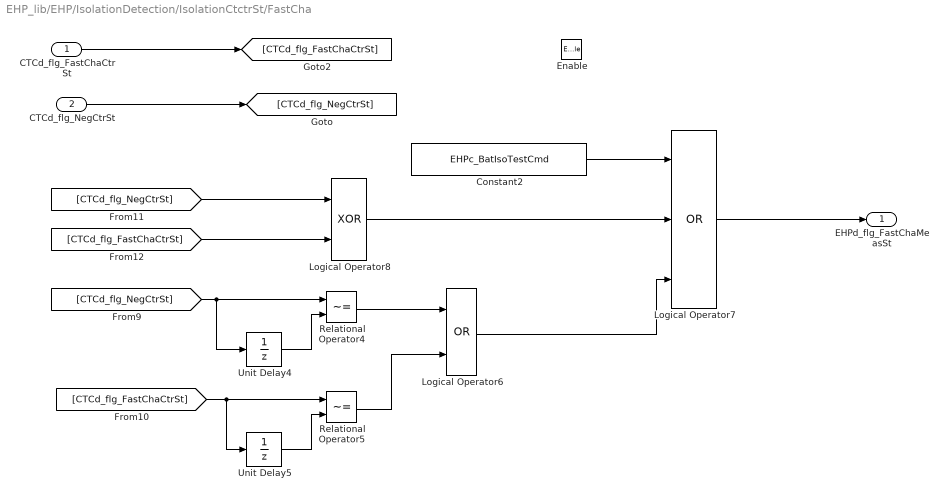
== system EHP_lib/EHP/IsolationDetection/IsolationCtctrSt/FastCha ==
  CTCd_flg_FastChaCtrSt : Inport  OutDataType=fixdt(1, 16)  OutScaling=2^0
  CTCd_flg_NegCtrSt : Inport  Port=2  OutDataType=fixdt(1, 16)  OutScaling=2^0
  Enable : EnablePort
  Constant2 : Constant  Value=EHPc_BatIsoTestCmd  OutDataTypeMode=boolean  OutDataType=fixdt(1, 16)  OutScaling=2^0  OutDataTypeStr=boolean
  Logical Operator6 : Logic  Operator=OR  AllPortsSameDT=off  OutDataTypeMode=boolean  LogicDataType=fixdt(0, 8)  OutDataTypeStr=boolean
  Logical Operator7 : Logic  Operator=OR  Inputs=3  AllPortsSameDT=off  OutDataTypeMode=boolean  LogicDataType=fixdt(0, 8)  OutDataTypeStr=boolean
  Logical Operator8 : Logic  Operator=XOR  AllPortsSameDT=off  OutDataTypeMode=boolean  LogicDataType=fixdt(0, 8)  OutDataTypeStr=boolean
  Relational Operator4 : RelationalOperator  Operator=~=  LogicOutDataTypeMode=boolean  LogicDataType=fixdt(0, 8)  OutDataTypeStr=boolean
  Relational Operator5 : RelationalOperator  Operator=~=  LogicOutDataTypeMode=boolean  LogicDataType=fixdt(0, 8)  OutDataTypeStr=boolean
  Unit Delay4 : UnitDelay  SampleTime=-1
  Unit Delay5 : UnitDelay  SampleTime=-1
  EHPd_flg_FastChaMeasSt : Outport  OutDataType=fixdt(1, 16)  OutScaling=2^0
  wires:
  Constant2/1 -> Logical Operator7/1
  Logical Operator7/1 -> EHPd_flg_FastChaMeasSt/1
  Logical Operator8/1 -> Logical Operator7/2
  Logical Operator6/1 -> Logical Operator7/3
  [CTCd_flg_FastChaCtrSt] -> Logical Operator8/2
  [CTCd_flg_NegCtrSt] -> Logical Operator8/1
  Relational Operator5/1 -> Logical Operator6/2
  Relational Operator4/1 -> Logical Operator6/1
  Unit Delay5/1 -> Relational Operator5/2
  [CTCd_flg_FastChaCtrSt] -> Relational Operator5/1, Unit Delay5/1
  Unit Delay4/1 -> Relational Operator4/2
  [CTCd_flg_NegCtrSt] -> Relational Operator4/1, Unit Delay4/1
  CTCd_flg_FastChaCtrSt/1 -> [CTCd_flg_FastChaCtrSt]
  CTCd_flg_NegCtrSt/1 -> [CTCd_flg_NegCtrSt]

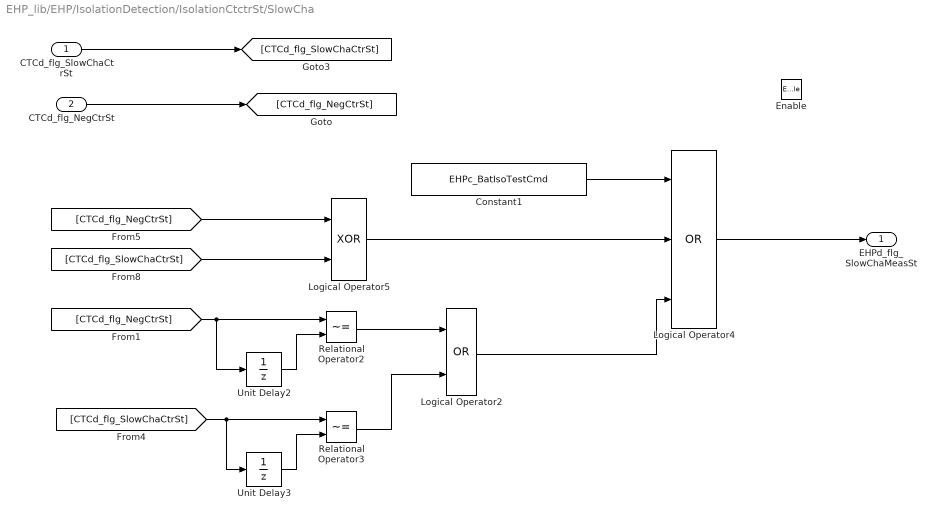
== system EHP_lib/EHP/IsolationDetection/IsolationCtctrSt/SlowCha ==
  CTCd_flg_SlowChaCtrSt : Inport  OutDataType=fixdt(1, 16)  OutScaling=2^0
  CTCd_flg_NegCtrSt : Inport  Port=2  OutDataType=fixdt(1, 16)  OutScaling=2^0
  Enable : EnablePort
  Constant1 : Constant  Value=EHPc_BatIsoTestCmd  OutDataTypeMode=boolean  OutDataType=fixdt(1, 16)  OutScaling=2^0  OutDataTypeStr=boolean
  Logical Operator2 : Logic  Operator=OR  AllPortsSameDT=off  OutDataTypeMode=boolean  LogicDataType=fixdt(0, 8)  OutDataTypeStr=boolean
  Logical Operator4 : Logic  Operator=OR  Inputs=3  AllPortsSameDT=off  OutDataTypeMode=boolean  LogicDataType=fixdt(0, 8)  OutDataTypeStr=boolean
  Logical Operator5 : Logic  Operator=XOR  AllPortsSameDT=off  OutDataTypeMode=boolean  LogicDataType=fixdt(0, 8)  OutDataTypeStr=boolean
  Relational Operator2 : RelationalOperator  Operator=~=  LogicOutDataTypeMode=boolean  LogicDataType=fixdt(0, 8)  OutDataTypeStr=boolean
  Relational Operator3 : RelationalOperator  Operator=~=  LogicOutDataTypeMode=boolean  LogicDataType=fixdt(0, 8)  OutDataTypeStr=boolean
  Unit Delay2 : UnitDelay  SampleTime=-1
  Unit Delay3 : UnitDelay  SampleTime=-1
  EHPd_flg_SlowChaMeasSt : Outport  OutDataType=fixdt(1, 16)  OutScaling=2^0
  wires:
  Constant1/1 -> Logical Operator4/1
  Logical Operator4/1 -> EHPd_flg_SlowChaMeasSt/1
  Logical Operator5/1 -> Logical Operator4/2
  Logical Operator2/1 -> Logical Operator4/3
  [CTCd_flg_SlowChaCtrSt] -> Logical Operator5/2
  [CTCd_flg_NegCtrSt] -> Logical Operator5/1
  Relational Operator3/1 -> Logical Operator2/2
  Relational Operator2/1 -> Logical Operator2/1
  Unit Delay3/1 -> Relational Operator3/2
  [CTCd_flg_SlowChaCtrSt] -> Relational Operator3/1, Unit Delay3/1
  Unit Delay2/1 -> Relational Operator2/2
  [CTCd_flg_NegCtrSt] -> Relational Operator2/1, Unit Delay2/1
  CTCd_flg_SlowChaCtrSt/1 -> [CTCd_flg_SlowChaCtrSt]
  CTCd_flg_NegCtrSt/1 -> [CTCd_flg_NegCtrSt]

== system EHP_lib/EHP/IsolationDetection/IsolationCalculation/IsolationCalculation/IslnClcnMeasV1>=V2 ==
  note: Calculation V1 >= V2:
  note: Ri=Ro(1+V2/V1)((V1-V1Line)/V1Line
  EHPd_v_PosCtrVol_chasis : Inport  OutDataType=fixdt(1, 16)  OutScaling=2^0
  EHPd_v_NegCtrVol_chasis : Inport  Port=2  OutDataType=fixdt(1, 16)  OutScaling=2^0
  EHPd_v_NegCtrVolR_chasis : Inport  Port=3  OutDataType=fixdt(1, 16)  OutScaling=2^0
  Enable : EnablePort
  Add : Sum  OutDataType=fixdt(1, 16)  OutScaling=2^-10  SaturateOnIntegerOverflow=on
  Add1 : Sum  Inputs=+-  OutDataType=fixdt(1, 16)  OutScaling=2^-10  SaturateOnIntegerOverflow=on
  Constant : Constant  OutDataTypeMode=single  OutDataType=fixdt(1, 16)  OutScaling=2^0  OutDataTypeStr=single
  Divide : Product  Inputs=*/  OutDataType=fixdt(1, 16)  OutScaling=2^-10  SaturateOnIntegerOverflow=on
  Divide1 : Product  Inputs=*/  OutDataType=fixdt(1, 16)  OutScaling=2^-10  SaturateOnIntegerOverflow=on
  Product : Product  OutDataType=fixdt(1, 16)  OutScaling=2^0  SaturateOnIntegerOverflow=on  RndMeth=Zero
  Product1 : Product  OutDataType=fixdt(1, 16)  OutScaling=2^0  SaturateOnIntegerOverflow=on  RndMeth=Zero
  Ro : Constant  Value=EHPc_r_ClcnRo  OutDataType=fixdt(1, 16)  OutScaling=2^0
  saturation : Defined_Functionality/saturation  SystemSampleTime=-1  upper_limit=10000000  lower_limit=1
      settings: AttributesFormatString=[UPPER_LIMIT=%<upper_limit>]\n[LOWER_LIMIT=%<lower_limit>]
  EHPd_r_PosIsoRes_raw : Outport  OutDataType=fixdt(1, 16)  OutScaling=2^0
  wires:
  saturation/1 -> EHPd_r_PosIsoRes_raw/1  "EHPd_r_PosIsoRes_raw"
  Constant/1 -> Add/2
  Ro/1 -> Product1/2
  Product1/1 -> saturation/1
  Product/1 -> Product1/1
  Divide1/1 -> Product/2
  Add/1 -> Product/1
  Add1/1 -> Divide1/1
  EHPd_v_NegCtrVolR_chasis/1 -> Divide1/2, Add1/2
  Divide/1 -> Add/1
  EHPd_v_NegCtrVol_chasis/1 -> Add1/1, Divide/2
  EHPd_v_PosCtrVol_chasis/1 -> Divide/1

== system EHP_lib/EHP/IsolationDetection/IsolationCalculation/IsolationCalculation/IslnClcnMeasV2>=V1 ==
  note: Calculation V2 > V1:
  note: Ri=Ro(1+V1/V2)((V2-V2Line)/V2Line)
  EHPd_v_NegCtrVol_chasis : Inport  OutDataType=fixdt(1, 16)  OutScaling=2^0
  EHPd_v_PosCtrVol_chasis : Inport  Port=2  OutDataType=fixdt(1, 16)  OutScaling=2^0
  EHPd_v_PosCtrVolR_chasis : Inport  Port=3  OutDataType=fixdt(1, 16)  OutScaling=2^0
  Enable : EnablePort
  Add : Sum  OutDataType=fixdt(1, 16)  OutScaling=2^-10
  Add1 : Sum  Inputs=+-  OutDataType=fixdt(1, 16)  OutScaling=2^-10
  Constant : Constant  OutDataTypeMode=single  OutDataType=fixdt(1, 16)  OutScaling=2^0  OutDataTypeStr=single
  Divide : Product  Inputs=*/  OutDataType=fixdt(1, 16)  OutScaling=2^-10
  Divide1 : Product  Inputs=*/  OutDataType=fixdt(1, 16)  OutScaling=2^-10
  Product : Product  OutDataType=fixdt(1, 16)  OutScaling=2^0  RndMeth=Zero
  Product1 : Product  OutDataType=fixdt(1, 16)  OutScaling=2^0  RndMeth=Zero
  Ro : Constant  Value=EHPc_r_ClcnRo  OutDataType=fixdt(1, 16)  OutScaling=2^0
  saturation : Defined_Functionality/saturation  SystemSampleTime=-1  upper_limit=10000000  lower_limit=1
      settings: AttributesFormatString=[UPPER_LIMIT=%<upper_limit>]\n[LOWER_LIMIT=%<lower_limit>]
  EHPd_r_NegIsoRes_raw : Outport  OutDataType=fixdt(1, 16)  OutScaling=2^0
  wires:
  Constant/1 -> Add/2
  saturation/1 -> EHPd_r_NegIsoRes_raw/1  "EHPd_r_NegIsoRes_raw"
  Ro/1 -> Product1/2
  Product1/1 -> saturation/1
  Product/1 -> Product1/1
  Divide1/1 -> Product/2
  Add/1 -> Product/1
  Add1/1 -> Divide1/1
  EHPd_v_PosCtrVolR_chasis/1 -> Divide1/2, Add1/2
  Divide/1 -> Add/1
  EHPd_v_PosCtrVol_chasis/1 -> Add1/1, Divide/2
  EHPd_v_NegCtrVol_chasis/1 -> Divide/1

== stateflow chart EHP/IsolationDetection/IsolationMeas/IslnMeas ==
  settings: description=|
      | $Author:Yan LiJuan$
      | $Date:2015/03/26$
      | $Revision:1.0$
  state Meas
    state State0
      EHPd_enum_StMeasIso=0;
    state UMeas
      state State1
        EHPd_enum_StMeasIso=1;
        du:EHPd_tm_MeasIso = EHPd_tm_MeasIso+10;
      state State2
        EHPd_enum_StMeasIso=2;
        du:EHPd_tm_MeasIso = EHPd_tm_MeasIso+10;
      state State4
        EHPd_enum_StMeasIso=4;
        du:EHPd_tm_MeasIso= EHPd_tm_MeasIso+10;
      state State3
        EHPd_enum_StMeasIso=3;
        du:EHPd_tm_MeasIso= EHPd_tm_MeasIso+10;
      state State5
        EHPd_enum_StMeasIso=5;
        du:EHPd_tm_MeasIso = EHPd_tm_MeasIso+10;
      state State6
        EHPd_enum_StMeasIso=6;
        du:EHPd_tm_MeasIso = EHPd_tm_MeasIso+10;
      state State7
        EHPd_enum_StMeasIso=7;
        du:EHPd_tm_MeasIso= EHPd_tm_MeasIso+10;
      state State8
        EHPd_enum_StMeasIso=8;
        du:EHPd_tm_MeasIso= EHPd_tm_MeasIso+10;
      (default) -> State1 : {EHPd_tm_MeasIso = 0;EHPd_enum_VoltCtrl = EHP_HvCtrl_St;EHP_TrigClcnAftMeas;}
      State1 -> State2 : [EHPd_tm_MeasIso >= EHPc_tm_MeasIso1_P]
          | {EHPd_tm_MeasIso = 0;EHPd_enum_VoltCtrl = EHP_HvPosCtrl_St;}
      State2 -> State3 : [EHPd_tm_MeasIso >= EHPc_tm_MeasIso2_P]
          | {EHPd_tm_MeasIso = 0;GET_HvPos=USample;EHPd_enum_VoltCtrl = EHP_HvCtrl_St;}
      State3 -> State4 : [EHPd_tm_MeasIso >= EHPc_tm_MeasIso3_P]
          | {EHPd_tm_MeasIso = 0;EHPd_enum_VoltCtrl = EHP_HvNegCtrl_St;}
      State4 -> State5 : [EHPd_tm_MeasIso >= EHPc_tm_MeasIso4_P]
          | {EHPd_tm_MeasIso = 0;GET_HvNeg=USample;EHPd_enum_VoltCtrl = EHP_HvCtrl_St;}
      State5 -> State6 : [EHPd_tm_MeasIso >= EHPc_tm_MeasIso5_P]
          | {EHPd_tm_MeasIso = 0;EHPd_enum_VoltCtrl = EHP_HvPosR0Ctrl_St;}
      State6 -> State7 : [EHPd_tm_MeasIso >= EHPc_tm_MeasIso6_P]
          | {EHPd_tm_MeasIso = 0;GET_HvPosR0=USample;EHPd_enum_VoltCtrl = EHP_HvCtrl_St;}
      State7 -> State8 : [EHPd_tm_MeasIso >= EHPc_tm_MeasIso7_P]
          | {EHPd_tm_MeasIso = 0;EHPd_enum_VoltCtrl = EHP_HvNegR0Ctrl_St;}
      State8 -> (junction 15) : [EHPd_tm_MeasIso >= EHPc_tm_MeasIso8_P]
          | {GET_HvNegR0=USample;EHPd_enum_VoltCtrl = EHP_HvCtrl_St;}
    State0 -> UMeas : [EHPd_flg_MeasStop==0]
    UMeas -> State0 : [EHPd_flg_MeasStop==1]
    (default) -> UMeas
  state Wait
    EHPd_enum_StMeasIso=9;
    du:
    EHPd_tm_Wait=EHPd_tm_Wait+10;
  Wait -> Meas : [EHPd_tm_Wait>=EHPc_tm_Wait_P]
  (junction 15) -> Wait : {EHPd_tm_Wait=0;EHP_TrigClcnAftMeas;}
  (default) -> Meas
  data: EHPc_tm_MeasIso1_P parameter uint16; EHPc_tm_MeasIso2_P parameter uint16; EHPc_tm_MeasIso3_P parameter uint16; EHPc_tm_MeasIso4_P parameter uint16; EHPc_tm_MeasIso5_P parameter uint16; EHPc_tm_MeasIso6_P parameter uint16; EHPc_tm_MeasIso7_P parameter uint16; EHPc_tm_MeasIso8_P parameter uint16; EHPd_flg_MeasStop input boolean; USample input single; GET_HvPos output single; GET_HvNeg output single; GET_HvPosR0 output single; GET_HvNegR0 output single; EHPd_enum_StMeasIso output uint8; EHPd_tm_Wait output uint16; EHPc_tm_Wait_P parameter uint16; EHPd_enum_VoltCtrl output uint8; EHP_HvCtrl_St parameter uint8; EHP_HvNegCtrl_St parameter uint8; EHP_HvNegR0Ctrl_St parameter uint8; EHP_HvPosCtrl_St parameter uint8; EHP_HvPosR0Ctrl_St parameter uint8; EHPd_tm_MeasIso output uint16
  events: EHP_TrigClcnAftMeas output EITHER_EDGE_EVENT
